simulink model "SiMoDronesMK"  (R2022a)
settings: Solver=FixedStepAuto  StartTime=0.0  StopTime=60  FixedStep=0.005  MaxStep=1e-3  MinStep=5e-5  RelTol=1e-5  AbsTol=1e-5  EnableMultiTasking=on
StopFcn:
  | save log.mat
  | [px4,optitrack,control,simulink]=traite_data_full('log.mat');
  | plot_data;
values from neighbouring files (symbols this model uses):
  aero =     [log.mat]
  drone =     [log.mat]
  dT_px4_udp = 0.02    [SimulationStartupScript.m]    (also in log.mat)
  dT_udp = 0.02    [SimulationStartupScript.m]    (also in log.mat)
  dT_udp_px4 = 0.02    [SimulationStartupScript.m]    (also in log.mat)
  Iload_UAVaxis = [0.00408625  0  0; 0  0.00408625  0; 0  0  8.625e-05]    [log.mat]
  init_state =     [log.mat]
  kpx = 1    [log.mat]
  kvx = 0.35    [log.mat]
  mass = 0.207    [log.mat]
  measure =     [log.mat]
  motor =     [log.mat]
  noisetrigger = 0    [log.mat]
  regul =     [log.mat]
  tdrop = 30    [SimulationStartupScript.m]    (also in log.mat)
  Te = 2e-2    (= 0.02)    [SimulationStartupScript.m]    (also in log.mat)
  th0 = 0.45    [log.mat]
  Ts_px4 = 5e-3    (= 0.005)    [SimulationStartupScript.m]    (also in log.mat)
undefined symbols (not defined in the file or in its folder): DiscIntNeverNeededParam, frame_t, gcbh, sigbuilder_block, sldrt_modeswitch, Standard_Devices, UDP_Protocol
libraries: simulink x11, orocomplib x9, vrlib x5, sldrtlib x4, sharedtransform x3, shared6dofsys x2, sharedutil x1, shared6dof x1, lib_isae_drones x1, simulink_need_slupdate x1, aerolibanimutils x1
(part 1 of 3)
Description:
  | SiMoDronesBE is an simulation environnement for ISAE drones dedicaded at the parrot + px4 bord drone.
settings Model: xpc_rtwmakecfg_data=_xpcnblib__xpcetherlib__xpcether8255xlib__xpcetherGbElib__xpciplib_  ExtModeTrigDuration=300000  Creator=Francois Defay  LastModifiedBy=fades
settings Model: ModifiedHistory=|
  | - Modification of measurement block and visualisation
  | - Some limitations of PWM have been added on the motor
settings SolverCC: AutoScaleAbsTol=off  ZeroCrossAlgorithm=Adaptive  AlgebraicLoopSolver=TrustRegion  AutoInsertRateTranBlk=on  InsertRTBMode=Always
settings DataIOCC: SaveFormat=Array  SaveOutput=off  SignalLogging=off  DSMLogging=off  SaveTime=off  ReturnWorkspaceOutputs=off
settings OptimizationCC: ExpressionDepthLimit=2147483647  LifeSpan=inf
settings DebuggingCC: UnderspecifiedInitializationDetection=Classic  MergeDetectMultiDrivingBlocksExec=none  IgnoredZcDiagnostic=none  SolverPrmCheckMsg=warning  MultiTaskDSMMsg=warning  UnconnectedInputMsg=warning  UnconnectedOutputMsg=warning  UnconnectedLineMsg=warning  AllowSymbolicDim=off  StateNameClashWarn=warning  SFUnexpectedBacktrackingDiag=warning  SFNoUnconditionalDefaultTransitionDiag=warning  SFExecutionAtInitializationDiag=none  SFMachineParentedDataDiag=warning  ArithmeticOperatorsInVariantConditions=warning
settings HardwareCC: ProdBitPerLong=64  ProdHWDeviceType=Intel->x86-64 (Linux 64)  TargetBitPerLong=64  TargetBitPerPointer=64  TargetIntDivRoundTo=Zero  TargetEndianess=LittleEndian  TargetWordSize=64  TargetHWDeviceType=Intel->x86-64
settings ModelReferenceCC: PropagateSignalLabelsOutOfModel=off
settings SFSimCC: SimUseLocalCustomCode=off  CustomCodeUndefinedFunction=UseInterfaceOnly
settings RTWCC: Description=Simulink Desktop Real-Time  SystemTargetFile=sldrt.tlc  TemplateMakefile=sldrt.tmf  RTWUseLocalCustomCode=off  RTWCompilerOptimization=on  DLArmComputeVersion=19.05
settings CodeAppCC: MaxIdLength=95  StateflowObjectComments=on
settings SimulinkDesktopRealTimeCC: TargetLibSuffix=_sldrt.a  TargetPreCompLibLocation=D:\toolbox\sldrt\lib\win64  TargetLangStandard=C89/C90 (ANSI)  SupportVariableSizeSignals=off
settings ConfigComp: CovMetricSettings=dw  CovSaveCumulativeToWorkspaceVar=on  CovSaveSingleToWorkspaceVar=on  CovExternalEMLEnable=off
settings SimscapeCC: SimscapeNormalizeSystem=off
settings ConfigurationSet: Description=SimMechanics 2G

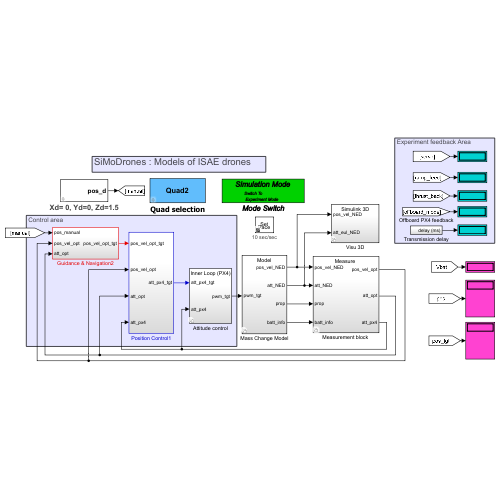
[thumbnail: Simulink's stored preview of the top-level diagram]
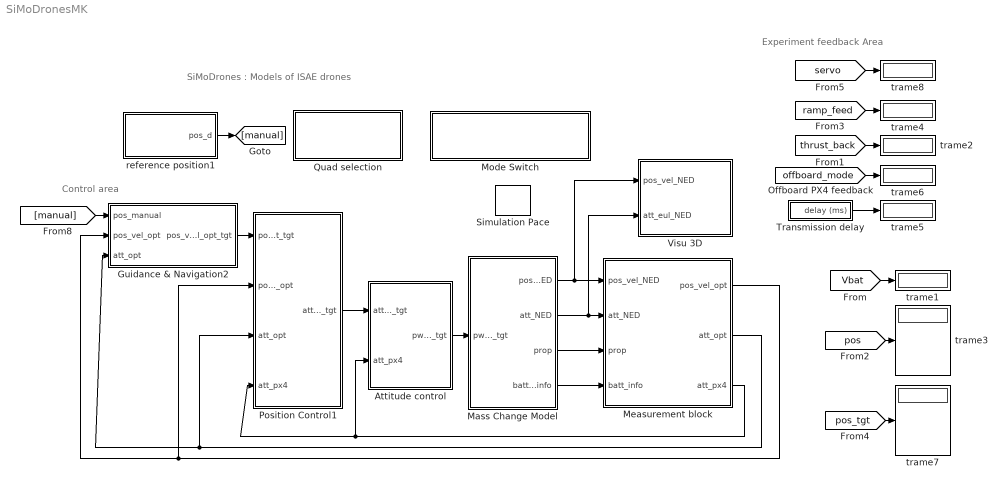
== system SiMoDronesMK ==
  note: Control area
  note: SiMoDrones : Models of ISAE drones
  note: Experiment feedback Area
   trame{1..8} (8 alike) : Display
  Attitude control : Subsystem  Variant=on
  Guidance & Navigation2 : Subsystem
  Mass Change Model : Subsystem  Variant=on
  "Measurement block " : Subsystem  Variant=on
  Mode Switch : Subsystem  LoadFcn=sldrt_modeswitch(gcbh, false)  mask(Mode Switch){}
      settings: OpenFcn=sldrt_modeswitch(gcbh, true)
      mask Display: text(0.5,0.8,'Simulation Mode', 'horizontalAlignment','center');text(0.5,0.5,'_{_{Switch To\newline Experiment Mode}}', 'horizontalAlignment','center','texmode','on');
  Position Control1 : Subsystem
  Quad selection : Subsystem  VariantControl=EXPERIMENT_MODE  mask{quadri_selected=QuadEdu_3}
      mask prompts: quadri_selected "Quadri"
      mask init:
      | assignin('base','quadri_selected', quadri_selected);
      | assignin('base','Quad1', Simulink.Variant('quadri_selected==1'));
      | assignin('base','Quad2', Simulink.Variant('quadri_selected==2'));
      | assignin('base','Quad3', Simulink.Variant('quadri_selected==3'));
      | 
      | if (quadri_selected == 1)
      |     set_param(gcbh, 'MaskDisplay', ...       'text(0.5,0.5,''Quad1'', ''horizontalAlignment'',''center'',''texmode'',''on'')');
      |        'disp(''Quad1'')');
      | elseif (quadri_selected == 2)
      |     set_param(gcbh, 'MaskDisplay', ...
      |        'disp(''MK6'')');
      | elseif (quadri_selected == 3)
      |     set_param(gcbh, 'MaskDisplay', ...
      |        'disp(''Quad2'')');
      | else
      |     set_param(gcbh, 'MaskDisplay', ...
      |        'disp(''No quad'')');
      | end
      mask TypeOptions quadri_selected: QuadEdu_1 | QuadEdu_2 | QuadEdu_3
      mask Display: disp('Quad2')
  Simulation Pace : aerolibanimutils/Simulation Pace  SimulationPace=10  SleepMode=MATLAB Thread  OutputPaceError=off  SampleTime=Te
      settings: AttributesFormatString=%<SimulationPace> sec/sec
  Transmission delay : Subsystem
  Visu 3D : Subsystem  Variant=on
  reference position1 : Subsystem  mask{xd=0, yd=0, zd=1.5}
      mask prompts: xd "X"; yd "Y"; zd "(-Z) Altitude"
      settings: AttributesFormatString=Xd= %<xd>, Yd=%<yd>, Zd=%<zd>
  wires:
  "Measurement block "/2(att_opt) -> Guidance & Navigation2/3(att_opt), Position Control1/3(att_opt)
  Mass Change Model/1(pos_vel_NED) -> "Measurement block "/1(pos_vel_NED), Visu 3D/1(pos_vel_NED)
  Mass Change Model/2(att_NED) -> "Measurement block "/2(att_NED), Visu 3D/2(att_eul_NED)
  Mass Change Model/3(prop) -> "Measurement block "/3(prop)
  Mass Change Model/4(batt_info) -> "Measurement block "/4(batt_info)
  "Measurement block "/1(pos_vel_opt) -> Guidance & Navigation2/2(pos_vel_opt), Position Control1/2(pos_vel_opt)
  Guidance & Navigation2/1(pos_vel_opt_tgt) -> Position Control1/1(pos_vel_opt_tgt)
  Position Control1/1(att_px4_tgt) -> Attitude control/1(att_px4_tgt)
  "Measurement block "/3(att_px4) -> Position Control1/4(att_px4), Attitude control/2(att_px4)
  Attitude control/1(pwm_tgt) -> Mass Change Model/1(pwm_tgt)
  [Vbat] -> " trame1"/1
  [thrust_back] -> " trame2"/1
  [pos] -> " trame3"/1
  [ramp_feed] -> " trame4"/1
  Transmission delay/1(delay (ms)) -> " trame5"/1
  [offboard_mode] -> " trame6"/1
  [pos_tgt] -> " trame7"/1
  [manual] -> Guidance & Navigation2/1(pos_manual)
  [servo] -> " trame8"/1
  reference position1/1(pos_d) -> [manual]

== system SiMoDronesMK/Attitude control ==
  att_px4_tgt : Inport
  att_px4 : Inport  Port=2
  Inner Loop (PX4) : Subsystem  VariantControl=SIMULATION_MODE
  Udp send : Subsystem  VariantControl=EXPERIMENT_MODE
  pwm_tgt : Outport

== system SiMoDronesMK/Guidance & Navigation2 ==
  pos_manual : Inport
  pos_vel_opt : Inport  Port=2
  att_opt : Inport  Port=3
  Bus Selector1 : BusSelector  OutputSignals=x,y,z
  Bus Selector2 : BusSelector  OutputSignals=vx,vy,vz
  Constant : Constant  Value=0
  Demux : Demux  Outputs=3
  Manual Switch3 : ManualSwitch  CurrentSetting=0
  Mux : Mux  Inputs=3
  Mux1 : Mux  Inputs=3
  Mux2 : Mux  Inputs=3
  Signal Builder : Subsystem  Tag=STV Subsys  LoadFcn=sigbuilder_block('load');  StartFcn=sigbuilder_block('start');  StopFcn=sigbuilder_block('stop');  ClipboardFcn=sigbuilder_block('clipboard');  mask(Sigbuilder block){tuvar=[0:10]}
      mask help: Simulink:masks:SigbuilderBlock_MD
      mask init:
      | if ~strcmp(get_param(bdroot(gcbh),'SimulationStatus'),'stopped') tuvar = sigbuilder_block('maskInit'); end
      settings: CopyFcn=sigbuilder_block('copy');  DeleteFcn=sigbuilder_block('delete');  ModelCloseFcn=sigbuilder_block('modelClose');  PreSaveFcn=sigbuilder_block('preSave');  PauseFcn=sigbuilder_block('pause');  ContinueFcn=sigbuilder_block('continue');  NameChangeFcn=sigbuilder_block('namechange');  OpenFcn=sigbuilder_block('open',[285 94 1149 508.25 ]);  CloseFcn=sigbuilder_block('close');
      mask Display: plot(0, 0, 100, 100,[2, 2, 32, 32, 2], [68, 8, 8, 68, 68],[32, 2], [38, 38], [32, 19, 2],[53, 60, 44], [32, 17, 17, 2],[16, 16, 31, 31]);txt = getActiveGroup(gcbh);text(2, 100, txt,'verticalAlignment', 'top');
  Subsystem : Subsystem
  Terminator : Terminator
  Terminator1 : Terminator
  To Workspace1 : ToWorkspace  VariableName=pos_tgt  SampleTime=Te
  To Workspace2 : ToWorkspace  VariableName=vit_tgt  SampleTime=Te
  pos_vel_opt_tgt : Outport  SampleTime=Te
  tag scope: pos_tgt=global
  wires:
  att_opt/1 -> Terminator/1
  Demux/3 -> Subsystem/3(Z_tgt)
  Demux/2 -> Subsystem/2(Y_tgt)
  Demux/1 -> Subsystem/1(X_tgt)
  Constant/1 -> Subsystem/4(Vx_tgt), Subsystem/6(Vz_tgt), Subsystem/5(Vy_tgt)
  Subsystem/1(pos_vel_opt_tgt) -> pos_vel_opt_tgt/1, Bus Selector2/1, Bus Selector1/1
  Mux1/1 -> To Workspace2/1
  Bus Selector2/3 -> Mux1/3  "<vz>"
  Bus Selector2/1 -> Mux1/1  "<vx>"
  Bus Selector2/2 -> Mux1/2  "<vy>"
  Mux/1 -> To Workspace1/1, [pos_tgt]
  Bus Selector1/3 -> Mux/3  "<z>"
  Bus Selector1/1 -> Mux/1  "<x>"
  Bus Selector1/2 -> Mux/2  "<y>"
  pos_manual/1 -> Manual Switch3/1
  Manual Switch3/1 -> Demux/1
  Mux2/1 -> Manual Switch3/2
  Signal Builder/2(Signal 2) -> Mux2/2
  Signal Builder/3(Signal 3) -> Mux2/3
  Signal Builder/1(Signal 1) -> Mux2/1
  pos_vel_opt/1 -> Terminator1/1

== system SiMoDronesMK/Mass Change Model ==
  pwm_tgt : Inport
  Model : Subsystem  VariantControl=SIMULATION_MODE
  Model disabled : Subsystem  VariantControl=EXPERIMENT_MODE
  pos_vel_NED : Outport
  att_NED : Outport  Port=2
  prop : Outport  Port=3
  batt_info : Outport  Port=4

== system SiMoDronesMK/Measurement block  ==
  pos_vel_NED : Inport
  att_NED : Inport  Port=2
  prop : Inport  Port=3
  batt_info : Inport  Port=4
  "Measure " : Subsystem  VariantControl=SIMULATION_MODE
  UDP link + Measure : Subsystem  VariantControl=EXPERIMENT_MODE
  pos_vel_opt : Outport
  att_opt : Outport  Port=2
  att_px4 : Outport  Port=3

== system SiMoDronesMK/Mode Switch ==
  mode : Constant  Value=0

== system SiMoDronesMK/Position Control1 ==
  pos_vel_opt_tgt : Inport
  pos_vel_opt : Inport  Port=2
  att_opt : Inport  Port=3
  att_px4 : Inport  Port=4  SampleTime=Te
  Bus Selector1 : BusSelector  OutputSignals=yaw
  Bus Selector3 : BusSelector  OutputSignals=yaw
  Delay6 : Delay  Commented=through  DelayLength=floor(dT_px4_udp/Te)  InitialCondition=0  SampleTime=Te
  Frame change : Subsystem
  Orocos Mapping : Subsystem
  X control : Subsystem
  Y  control : Subsystem
  Z  control : Subsystem
  psi_opt_tgt : Constant  Value=0
  px4 yaw compensation : Subsystem
  att_px4_tgt : Outport
  wires:
  Orocos Mapping/1(att_px4_tgt) -> att_px4_tgt/1
  px4 yaw compensation/1(yaw_tgt_px4) -> Orocos Mapping/3(yaw)
  pos_vel_opt_tgt/1 -> Y  control/1(pos_vel_opt_tgt), X control/1(pos_vel_opt_tgt), Z  control/1(pos_vel_opt_tgt)
  att_opt/1 -> Bus Selector3/1
  att_px4/1 -> Delay6/1
  Bus Selector3/1 -> px4 yaw compensation/1(psi_opt), Frame change/3(psi)  "<yaw>"
  psi_opt_tgt/1 -> px4 yaw compensation/2(psi_opt_tgt)
  Bus Selector1/1 -> px4 yaw compensation/3(psi_px4)  "<yaw>"
  Delay6/1 -> Bus Selector1/1
  pos_vel_opt/1 -> Y  control/2(pos_vel_opt), X control/2(pos_vel_opt), Z  control/2(pos_vel_opt)
  X control/1(Pitch_tgt) -> Frame change/2(pitch_tgt)
  Y  control/1(Roll_tgt) -> Frame change/1(roll_tgt)
  Z  control/1(Thrust[0..1]) -> Orocos Mapping/4(thrust [0..1])
  Frame change/2(pitch_command) -> Orocos Mapping/2(pitch)
  Frame change/1(roll_command) -> Orocos Mapping/1(roll)

== system SiMoDronesMK/Quad selection ==

== system SiMoDronesMK/Transmission delay ==
  Add : Sum  Inputs=+-
  Data Type Conversion1 : DataTypeConversion  OutDataTypeStr=double  SaturateOnIntegerOverflow=off  LockScale=on
  Gain1 : Gain  Gain=10
  delay (ms) : Outport
  wires:
  [ramp_feed] -> Add/2
  [ramp_out] -> Add/1
  Gain1/1 -> delay (ms)/1
  Add/1 -> Data Type Conversion1/1
  Data Type Conversion1/1 -> Gain1/1

== system SiMoDronesMK/Visu 3D ==
  pos_vel_NED : Inport
  att_eul_NED : Inport  Port=2
  3D disabled : Subsystem  VariantControl=EXPERIMENT_MODE
  Simulink 3D : Subsystem  VariantControl=SIMULATION_MODE

== system SiMoDronesMK/reference position1 ==
  Constant1 : Constant  Value=xd  SampleTime=Te
  Constant2 : Constant  Value=yd  SampleTime=Te
  Constant4 : Constant  Value=zd  SampleTime=Te
  Gain : Gain  Gain=-1
  Mux : Mux  Inputs=3
  pos_d : Outport
  wires:
  Constant1/1 -> Mux/1
  Constant2/1 -> Mux/2
  Constant4/1 -> Gain/1
  Mux/1 -> pos_d/1
  Gain/1 -> Mux/3

== system SiMoDronesMK/Attitude control/Inner Loop (PX4) ==
  att_px4_tgt : Inport
  att_px4 : Inport  Port=2
  Attitude Control Actuators (PID-PX4) : Subsystem  VariantControl=SIMULATION_SIMULINK  mask(PX4 attitude controller){Kp_att=regul.px4.Kp_att, yaw_ff=regul.px4.Yaw_ff, yaw_sp_move_rate=regul.px4.Yaw_move_rate, mc_rate_max=regul.px4.max_rate, Kp_rate=regul.px4.Kp_rate, Ki_rate=regul.px4.Ki_rate, Kd_rate=regul.px4.Kd_rate, ff_rate=regul.px4.ff_rate}
      mask prompts: Kp_att "Proportional gains"; yaw_ff "Yaw feedforward gain"; yaw_sp_move_rate "Yaw move rate"; mc_rate_max "Max rate output (deg/s)"; Kp_rate "Proportional gains"; Ki_rate "Integral gains"; Kd_rate "Derivative gains"; ff_rate "Feedforward gains"
      mask DialogControl Container4 Prompt: MC Attitude control
      mask DialogControl Container12 Prompt: MC Attitude rate control
  Mixer_Quad_X : Subsystem  mask(Mixer Quad X){}
      mask help:
      | Mixer used by a PX4 configured with a Quad X airframe.
      |
      | It takes in the the actuators target (normalized roll, pitch, yaw [-1..1], thrust [0..1]) and mixes them with the Quad X mixer matrix into 4 motors PWM ([0..1]).
      mask DialogControl Container2 Prompt: Parameters
  To Workspace3 : ToWorkspace  Commented=on  VariableName=pwm_target  SampleTime=Te
  pwm_tgt : Outport
  wires:
  att_px4/1 -> Attitude Control Actuators (PID-PX4)/2(att_eul_PX4)
  Attitude Control Actuators (PID-PX4)/1(actuator_target) -> Mixer_Quad_X/1(actuators_tgt)
  Mixer_Quad_X/1(pwm_out) -> pwm_tgt/1, To Workspace3/1
  att_px4_tgt/1 -> Attitude Control Actuators (PID-PX4)/1(att_eul_tgt)

== system SiMoDronesMK/Attitude control/Udp send ==
  att_px4_tgt : Inport
  Bus Selector : BusSelector  OutputSignals=roll,pitch,yaw,thrust
  Constant : Constant  OutDataTypeStr=int16  SampleTime=Te
  Counter Free-Running : simulink/Sources/Counter Free-Running  NumBits=16  tsamp=Te
  Mux : Mux
  To Workspace1 : ToWorkspace  VariableName=att_tgt_px4  SampleTime=Te
  To Workspace3 : ToWorkspace  VariableName=ramp1  SampleTime=Te
  send_udp : Subsystem  Variant=on
  udpSend : MATLAB Function  TreatAsAtomicUnit=on
  tag scope: ramp_out=global
  wires:
  att_px4_tgt/1 -> Bus Selector/1, udpSend/1(att_eul_tgt)
  Constant/1 -> udpSend/2(simulink_out_mode)
  Counter Free-Running/1 -> [ramp_out], To Workspace3/1, udpSend/3(ramp)
  [offboard_mode] -> udpSend/4(simulink_activated)
  udpSend/1(floats) -> send_udp/1(float)
  udpSend/2(integers) -> send_udp/2(Int)
  Mux/1 -> To Workspace1/1
  Bus Selector/4 -> Mux/4  "<thrust>"
  Bus Selector/3 -> Mux/3  "<yaw>"
  Bus Selector/2 -> Mux/2  "<pitch>"
  Bus Selector/1 -> Mux/1  "<roll>"

== system SiMoDronesMK/Guidance & Navigation2/Signal Builder ==
  Demux : Demux  Tag=STV Demux  Outputs=3
      settings: DisplayOption=none
  FromWs : FromWorkspace  Tag=STV FromWs  VariableName=tuvar
      SigBuilderData=|
      | common.afterFinalStr = 'Extrapolate'
      | common.sampleTime = 0
      | dataSet.timeRange = [0 60]
      | dataSet.name = 'Group 1'
      | sbobj.Groups.Name = 'Group 1'
      | sbobj.Groups.Signals(1).Name = 'Signal 1'
      | sbobj.Groups.Signals(1).XData = [0 25 60]
      | sbobj.Groups.Signals(1).YData = [0 0 0]
      | sbobj.Groups.Signals(2).Name = 'Signal 2'
      | sbobj.Groups.Signals(2).XData = [0 5 60]
      | sbobj.Groups.Signals(2).YData = [0 0 0]
      | sbobj.Groups.Signals(3).Name = 'Signal 3'
      | sbobj.Groups.Signals(3).XData = [0 3.45 5 5 15 15 22 22 38 38 45 45 52 55 60]
      | sbobj.Groups.Signals(3).YData = [0 0 -0.75 -0.7 -0.7 -2.15 -2.15 -1.5 -1.5 -2 -2 -1.5 -1.5 0 0]
      | sbobj.Groups.TimeRange = [0 60]
  Signal 1 : Outport  Tag=STV Outport
  Signal 2 : Outport  Tag=STV Outport  Port=2
  Signal 3 : Outport  Tag=STV Outport  Port=3
  wires:
  FromWs/1 -> Demux/1
  Demux/1 -> Signal 1/1
  Demux/2 -> Signal 2/1
  Demux/3 -> Signal 3/1

== system SiMoDronesMK/Guidance & Navigation2/Subsystem ==
  X_tgt : Inport
  Y_tgt : Inport  Port=2
  Z_tgt : Inport  Port=3
  Vx_tgt : Inport  Port=4
  Vy_tgt : Inport  Port=5
  Vz_tgt : Inport  Port=6
  Constant1 : Constant  Value=frame_t.LOCAL_NED
  OROCOS TYPE pos_vel : orocomplib/OROCOS TYPE pos_vel
      settings: SourceProductName=Orocos Component Target
  pos_vel_opt_tgt : Outport
  wires:
  Vx_tgt/1 -> OROCOS TYPE pos_vel/6
  Vz_tgt/1 -> OROCOS TYPE pos_vel/8
  ? -> OROCOS TYPE pos_vel/1
  Vy_tgt/1 -> OROCOS TYPE pos_vel/7
  Z_tgt/1 -> OROCOS TYPE pos_vel/5
  Y_tgt/1 -> OROCOS TYPE pos_vel/4
  X_tgt/1 -> OROCOS TYPE pos_vel/3
  Constant1/1 -> OROCOS TYPE pos_vel/2
  OROCOS TYPE pos_vel/1 -> pos_vel_opt_tgt/1

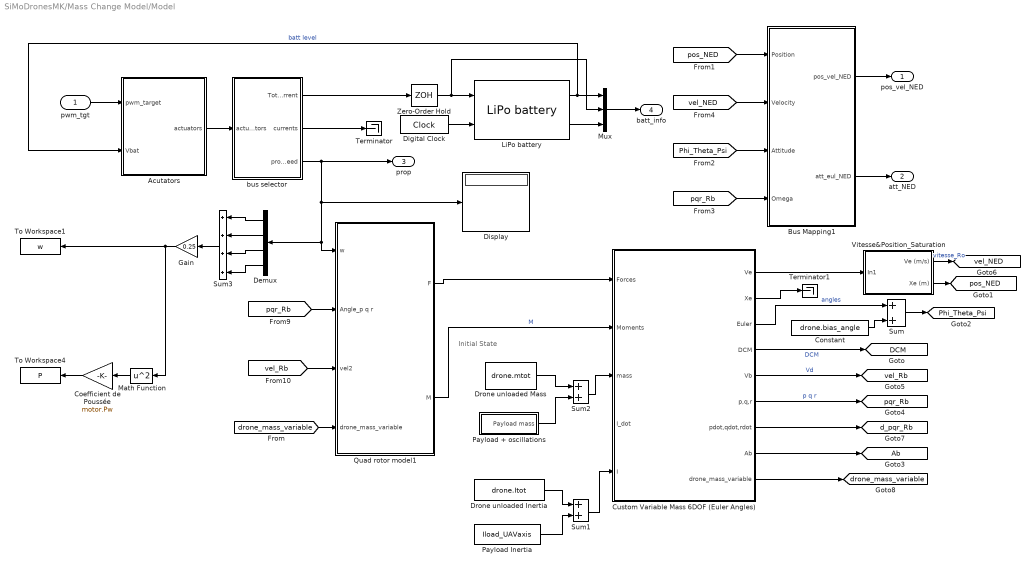
== system SiMoDronesMK/Mass Change Model/Model ==
  note: Initial State
  pwm_tgt : Inport
  Acutators : Subsystem
  Bus Mapping1 : Subsystem
  Coefficient de Poussée : Gain  Gain=motor.Pw
  Constant : Constant  Value=drone.bias_angle
  Custom Variable Mass 6DOF (Euler Angles) : Subsystem  AncestorBlock=shared6dof/6DOF (Euler Angles)  mask(6DOF EoM (Body Axis)){units=Metric (MKS), mtype=Custom Variable, rep=Euler Angles, xme_0=init_state.Pterre0, Vm_0=init_state.Vuvw0, eul_0=init_state.Angles0, pm_0=init_state.pqr0, mass_0=1.0, mass_e=0.5, mass_f=2.0, inertia=eye(3), inertia_e=eye(3), inertia_f=2*eye(3), k_quat=1.0, vre_flag=off, abi_flag=off, aMode=0, xme_statename='', Vm_statename='', eul_statename='', quat_statename='', pm_statename='', mass_statename=''}
      mask prompts: units "shared_aeroblks:sharedaeroblk6dofbody:block6DOFEoMBodyAxisParamUnits"; mtype "shared_aeroblks:sharedaeroblk6dofbody:block6DOFEoMBodyAxisParamMasstype"; rep "shared_aeroblks:sharedaeroblk6dofbody:block6DOFEoMBodyAxisParamRepresentation"; xme_0 "shared_aeroblks:sharedaeroblk6dofbody:block6DOFEoMBodyAxisParamInitialpositionininertialaxesXeYeZe"; Vm_0 "shared_aeroblks:sharedaeroblk6dofbody:block6DOFEoMBodyAxisParamInitialvelocityinbodyaxesUvw"; eul_0 "shared_aeroblks:sharedaeroblk6dofbody:block6DOFEoMBodyAxisParamInitialEulerorientationrollpitchyaw"; pm_0 "shared_aeroblks:sharedaeroblk6dofbody:block6DOFEoMBodyAxisParamInitialbodyrotationratespqr"; mass_0 "shared_aeroblks:sharedaeroblk6dofbody:block6DOFEoMBodyAxisParamInitialmass"; mass_e "shared_aeroblks:sharedaeroblk6dofbody:block6DOFEoMBodyAxisParamEmptymass"; mass_f "shared_aeroblks:sharedaeroblk6dofbody:block6DOFEoMBodyAxisParamFullmass"; inertia "shared_aeroblks:sharedaeroblk6dofbody:block6DOFEoMBodyAxisParamInertia"; inertia_e "shared_aeroblks:sharedaeroblk6dofbody:block6DOFEoMBodyAxisParamEmptyinertiamatrix"; inertia_f "shared_aeroblks:sharedaeroblk6dofbody:block6DOFEoMBodyAxisParamFullinertiamatrix"; k_quat "shared_aeroblks:sharedaeroblk6dofbody:block6DOFEoMBodyAxisParamGainforquaternionnormalization"; vre_flag "shared_aeroblks:sharedaeroblk6dofbody:block6DOFEoMBodyAxisParamIncludemassflowrelativevelocity"; abi_flag "shared_aeroblks:sharedaeroblk6dofbody:inertialAccelFlag"; xme_statename "shared_aeroblks:sharedaeroblk6dofbody:block6DOFEoMStateNamePosition"; Vm_statename "shared_aeroblks:sharedaeroblk6dofbody:block6DOFEoMStateNameVelocity"; eul_statename "shared_aeroblks:sharedaeroblk6dofbody:block6DOFEoMStateNameEulerAngles"; quat_statename "shared_aeroblks:sharedaeroblk6dofbody:block6DOFEoMStateNameQuaternions"; pm_statename "shared_aeroblks:sharedaeroblk6dofbody:block6DOFEoMStateNameRotationRates"; mass_statename "shared_aeroblks:sharedaeroblk6dofbody:block6DOFEoMStateNameMass"
      mask help: shared_aeroblks:sharedaeroblk6dofbody:block6DOFEoMBodyAxisDesc
      mask init:
      | if aerosharedtest(gcb)
      |     ports=aerosharedicon('shared6dofbody','icon');
      | else
      |     ports=sharedautoicon('shared6dofbody','icon');
      | end
      mask Help: eval('aerosharedhelp(''custom_variable_mass_sixdof_euler_angles'')');
      mask TypeOptions units: shared_aeroblks:sharedaeroblk6dofbody:block6DOFEoMBodyAxisParamComboMetricMKS | shared_aeroblks:sharedaeroblk6dofbody:block6DOFEoMBodyAxisParamComboEnglishVelocityinfts | shared_aeroblks:sharedaeroblk6dofbody:block6DOFEoMBodyAxisParamComboEnglishVelocityinkts
      mask TypeOptions mtype: shared_aeroblks:sharedaeroblk6dofbody:block6DOFEoMBodyAxisParamComboFixed | shared_aeroblks:sharedaeroblk6dofbody:block6DOFEoMBodyAxisParamComboSimpleVariable | shared_aeroblks:sharedaeroblk6dofbody:block6DOFEoMBodyAxisParamComboCustomVariable
      mask Callback mtype:
      | if aerosharedtest(gcb) && builtin('license','test','aerospace_blockset')
      |     aerosharedicon('shared6dofbody');
      | else
      |     sharedautoicon('shared6dofbody');
      | end
      mask TypeOptions rep: shared_aeroblks:sharedaeroblk6dofbody:block6DOFEoMBodyAxisParamComboEulerAngles | shared_aeroblks:sharedaeroblk6dofbody:block6DOFEoMBodyAxisParamComboQuaternion
      mask Callback rep:
      | if aerosharedtest(gcb) && builtin('license','test','aerospace_blockset')
      |     aerosharedicon('shared6dofbody');
      | else
      |     sharedautoicon('shared6dofbody');
      | end
      mask DialogControl Container4 Prompt: shared_aeroblks:sharedaeroblk6dofbody:block6DOFEoMParamTab
      mask DialogControl units Prompt: Units:
      mask DialogControl mtype Prompt: Mass type:
      mask DialogControl rep Prompt: Representation:
      mask DialogControl xme_0 Prompt: Initial position in inertial axes [Xe,Ye,Ze]:
      mask DialogControl Vm_0 Prompt: Initial velocity in body axes [U,v,w]:
      mask DialogControl eul_0 Prompt: Initial Euler orientation [roll, pitch, yaw]:
      mask DialogControl pm_0 Prompt: Initial body rotation rates [p,q,r]:
      mask DialogControl mass_0 Prompt: Initial mass:
      mask DialogControl mass_e Prompt: Empty mass:
      mask DialogControl mass_f Prompt: Full mass:
      mask DialogControl inertia Prompt: Inertia:
      mask DialogControl inertia_e Prompt: Empty inertia matrix:
      mask DialogControl inertia_f Prompt: Full inertia matrix:
      mask DialogControl k_quat Prompt: Gain for quaternion normalization:
      mask DialogControl vre_flag Prompt: Include mass flow relative velocity
      mask DialogControl abi_flag Prompt: Include inertial acceleration
      mask DialogControl Container6 Prompt: shared_aeroblks:sharedaeroblk6dofbody:block6DOFEoMStateAttributesTab
      mask DialogControl Container7 Prompt: shared_aeroblks:sharedaeroblk6dofbody:block6DOFEoMStateNamesGroup
      mask DialogControl xme_statename Prompt: Position: e.g., {'Xe', 'Ye', 'Ze'}
      mask DialogControl Vm_statename Prompt: Velocity: e.g., {'U', 'v', 'w'}
      mask DialogControl eul_statename Prompt: Euler rotation angles: e.g., {'phi', 'theta', 'psi'}
      mask DialogControl quat_statename Prompt: Quaternion vector: e.g., {'qr', 'qi', 'qj', 'qk'}
      mask DialogControl pm_statename Prompt: Body rotation rates: e.g., {'p', 'q', 'r'}
      mask DialogControl mass_statename Prompt: Mass: e.g., 'mass'
      mask Display:
      | port_label(ports(1).type,ports(1).port,ports(1).txt,'texmode','on');
      | port_label(ports(2).type,ports(2).port,ports(2).txt,'texmode','on');
      | port_label(ports(3).type,ports(3).port,ports(3).txt,'texmode','on');
      | port_label(ports(4).type,ports(4).port,ports(4).txt,'texmode','on');
      | port_label(ports(5).type,ports(5).port,ports(5).txt,'texmode','on');
      | port_label(ports(6).type,ports(6).port,ports(6).txt,'texmode','on');
      | port_label(ports(7).type,ports(7).port,ports(7).txt,'texmode','on');
      | port_label(ports(8).type,ports(8).port,ports(8).txt,'texmode','on');
      | port_label(ports(9).type,ports(9).port,ports(9).txt,'texmode','on');
      | port_label(ports(10).type,ports(10).port,ports(10).txt,'texmode','on');
      | port_label(ports(11).type,ports(11).port,ports(11).txt,'texmode','on');
      | port_label(ports(12).type,ports(12).port,ports(12).txt,'texmode','on');
      | port_label(ports(13).type,ports(13).port,ports(13).txt,'texmode','on');
      | port_label(ports(14).type,ports(14).port,ports(14).txt,'texmode','on');
      | port_label(ports(15).type,ports(15).port,ports(15).txt,'texmode','on');
      | port_label(ports(16).type,ports(16).port,ports(16).txt,'texmode','on');
      | port_label(ports(17).type,ports(17).port,ports(17).txt,'texmode','on');
  Demux : Demux
  Digital Clock : DigitalClock  SampleTime=Te
  Display : Display
  Drone unloaded Inertia : Constant  Value=drone.Itot
  Drone unloaded Mass : Constant  Value=drone.mtot
  Gain : Gain  Gain=0.25
  LiPo battery : lib_isae_drones/LiPo battery  nb_elements=batt.nb_element  capacity=batt.capacity  initial_voltage=batt.initial_voltage  internal_resistance=batt.internal_resistance
      settings: SourceProductName=ISAE drones
  Math Function : Math  Operator=square  SignedPower=on
  Mux : Mux  Inputs=3
  "Payload + oscillations " : Subsystem
  Payload Inertia : Constant  Value=Iload_UAVaxis
  Quad rotor model1 : Subsystem  mask{Pw=motor.Pw, L=drone.length_arm, Mw=motor.Mw, mtot=drone.mtot, rho=aero.rho, S_drag_uvw=aero.S_trainee_uvw, C_drag=aero.C_trainee, g=aero.g, C_trainee=0, S_trainee_pqr=0}
      mask prompts: Pw "Thrust factor"; L "Length of the arm"; Mw "Torque coefficient"; mtot "Total mass"; rho "Air density"; S_drag_uvw "Drag Surface"; C_drag "Drag coefficient"; g "Gravity constant"; C_trainee "rotationnal drag coef"; S_trainee_pqr "rotationnal drag surface"
  Sum : Sum
  Sum1 : Sum
  Sum2 : Sum
  Sum3 : Sum  Inputs=++++
  Terminator : Terminator
  Terminator1 : Terminator
  To Workspace1 : ToWorkspace  VariableName=w  SampleTime=Te
  To Workspace4 : ToWorkspace  VariableName=P  SampleTime=Te
  Vitesse&Position_Saturation : Subsystem
  Zero-Order Hold : ZeroOrderHold  SampleTime=Te
  bus selector : Subsystem
  pos_vel_NED : Outport
  att_NED : Outport  Port=2
  prop : Outport  Port=3
  batt_info : Outport  Port=4
  tag scope: Ab=global, DCM=global, Phi_Theta_Psi=global, d_pqr_Rb=global, drone_mass_variable=global, pos_NED=global, pqr_Rb=global, vel_NED=global, vel_Rb=global
  wires:
  Vitesse&Position_Saturation/1(Ve (m/s)) -> [vel_NED]  "vitesse_Ro"
  Custom Variable Mass 6DOF (Euler Angles)/8(Ab) -> [Ab]
  Custom Variable Mass 6DOF (Euler Angles)/5(Vb) -> [vel_Rb]  "Vd"
  Custom Variable Mass 6DOF (Euler Angles)/4(DCM) -> [DCM]  "DCM"
  Custom Variable Mass 6DOF (Euler Angles)/3(Euler) -> Sum/1  "angles"
  Custom Variable Mass 6DOF (Euler Angles)/1(Ve) -> Vitesse&Position_Saturation/1(In1)
  Custom Variable Mass 6DOF (Euler Angles)/2(Xe) -> Terminator1/1
  Custom Variable Mass 6DOF (Euler Angles)/6(p,q,r) -> [pqr_Rb]  "p q r"
  Custom Variable Mass 6DOF (Euler Angles)/7(pdot,qdot,rdot) -> [d_pqr_Rb]
  bus selector/3(prop speed) -> prop/1, Demux/1, Quad rotor model1/1(w), Display/1
  [pqr_Rb] -> Quad rotor model1/2(Angle_p q r)
  Mux/1 -> batt_info/1
  bus selector/2(currents) -> Terminator/1
  bus selector/1(Total current) -> Zero-Order Hold/1
  LiPo battery/2 -> Mux/3
  Digital Clock/1 -> LiPo battery/2
  LiPo battery/1 -> Acutators/2(Vbat), Mux/1  "batt level"
  pwm_tgt/1 -> Acutators/1(pwm_target)
  Acutators/1(actuators) -> bus selector/1(actuators)
  [pos_NED] -> Bus Mapping1/1(Position)
  [vel_NED] -> Bus Mapping1/2(Velocity)
  [pqr_Rb] -> Bus Mapping1/4(Omega)
  [Phi_Theta_Psi] -> Bus Mapping1/3(Attitude)
  Bus Mapping1/2(att_eul_NED) -> att_NED/1
  Bus Mapping1/1(pos_vel_NED) -> pos_vel_NED/1
  [vel_Rb] -> Quad rotor model1/3(vel2)
  Sum/1 -> [Phi_Theta_Psi]
  Constant/1 -> Sum/2
  Vitesse&Position_Saturation/2(Xe (m)) -> [pos_NED]
  Quad rotor model1/1(F) -> Custom Variable Mass 6DOF (Euler Angles)/1(Forces)
  Quad rotor model1/2(M) -> Custom Variable Mass 6DOF (Euler Angles)/2(Moments)  "M"
  Drone unloaded Mass/1 -> Sum2/1
  Custom Variable Mass 6DOF (Euler Angles)/9(drone_mass_variable) -> [drone_mass_variable]
  Drone unloaded Inertia/1 -> Sum1/1
  Sum1/1 -> Custom Variable Mass 6DOF (Euler Angles)/5(I)
  Sum2/1 -> Custom Variable Mass 6DOF (Euler Angles)/3(mass)
  "Payload + oscillations "/1(Payload mass) -> Sum2/2
  Payload Inertia/1 -> Sum1/2
  [drone_mass_variable] -> Quad rotor model1/4(drone_mass_variable)
  Demux/1 -> Sum3/1
  Demux/2 -> Sum3/2
  Demux/3 -> Sum3/3
  Demux/4 -> Sum3/4
  Sum3/1 -> Gain/1
  Gain/1 -> To Workspace1/1, Math Function/1
  Math Function/1 -> Coefficient de Poussée/1
  Coefficient de Poussée/1 -> To Workspace4/1
  Zero-Order Hold/1 -> Mux/2, LiPo battery/1

== system SiMoDronesMK/Mass Change Model/Model disabled ==

== system SiMoDronesMK/Measurement block /Measure  ==
  pos_vel_NED : Inport
  att_NED : Inport  Port=2
  prop : Inport  Port=3
  batt_info : Inport  Port=4
  Band-Limited White Noise4 : simulink/Sources/Band-Limited White Noise  Cov=[measure.noise_power_propellers]  Ts=Te  seed=[23341]
  Clock : Clock
  Delay2 : Delay  DelayLength=floor(dT_px4_udp/Te)  InitialCondition=0  SampleTime=Te
  Demux : Demux  Outputs=2
  Sum4 : Sum  Inputs=++|
  Terminator : Terminator
  To Workspace5 : ToWorkspace  VariableName=batt_info  SampleTime=Te
  To Workspace6 : ToWorkspace  Commented=on  VariableName=prop_mes  SampleTime=Te
  To Workspace8 : ToWorkspace  VariableName=time_simu  SampleTime=Te
  Zero-Order Hold8 : ZeroOrderHold  SampleTime=0.5
  optitrack : Subsystem
  px4 : Subsystem
  pos_vel_opt : Outport
  att_opt : Outport  Port=2
  att_px4 : Outport  Port=3
  tag scope: Vbat=global, pos=global
  wires:
  optitrack/2(att_eul_optitrack) -> att_opt/1
  optitrack/1(pos_vel_optitrack) -> pos_vel_opt/1
  pos_vel_NED/1 -> Demux/1, optitrack/1(pos_vel_NED)
  px4/1(att_eul_px4) -> att_px4/1
  Delay2/1 -> Sum4/2
  Zero-Order Hold8/1 -> [Vbat], To Workspace5/1
  Clock/1 -> To Workspace8/1
  batt_info/1 -> Zero-Order Hold8/1
  att_NED/1 -> px4/1(att_eul_NED), optitrack/2(att_eul_NED)
  prop/1 -> Delay2/1
  Band-Limited White Noise4/1 -> Sum4/1
  Sum4/1 -> To Workspace6/1, Terminator/1  "prop_mes"
  Demux/1 -> [pos]

== system SiMoDronesMK/Measurement block /UDP link + Measure ==
  Mesure : Subsystem
  UDP link : Subsystem
  pos_vel_opt : Outport
  att_px4 : Outport  Port=2
  att_opt : Outport  Port=3
  wires:
  Mesure/1(pos_vel_optitrack) -> pos_vel_opt/1
  Mesure/2(att_eul_optitrack) -> att_opt/1
  Mesure/3(att_eul_px4_) -> att_px4/1
  UDP link/2(att_eul_optitrack) -> Mesure/2(att_eul_opti)
  UDP link/1(pos_vel_optitrack) -> Mesure/1(pos_vel_opti)
  UDP link/3(att_eul_px4) -> Mesure/3(att_eul_px4)

== system SiMoDronesMK/Position Control1/Frame change ==
  roll_tgt : Inport
  pitch_tgt : Inport  Port=2
  psi : Inport  Port=3
  Add : Sum
  Add1 : Sum
  Gain1 : Gain  Gain=-1
  Product{,1..3} (4 alike) : Product
  Saturation : Saturate  UpperLimit=0.3  LowerLimit=-0.3
  Saturation1 : Saturate  UpperLimit=0.3  LowerLimit=-0.3
  Trigonometric Function : Trigonometry
  Trigonometric Function1 : Trigonometry  Operator=cos
  Trigonometric Function2 : Trigonometry
  Trigonometric Function3 : Trigonometry  Operator=cos
  roll_command : Outport
  pitch_command : Outport  Port=2
  wires:
  Gain1/1 -> Product/1
  Add1/1 -> Saturation1/1
  Product3/1 -> Add1/2
  Trigonometric Function1/1 -> Product3/1
  Product2/1 -> Add1/1
  Trigonometric Function2/1 -> Product2/1
  psi/1 -> Trigonometric Function/1, Trigonometric Function3/1, Trigonometric Function2/1, Trigonometric Function1/1
  Add/1 -> Saturation/1
  Product1/1 -> Add/2
  pitch_tgt/1 -> Product1/2, Product2/2
  Trigonometric Function3/1 -> Product1/1
  Product/1 -> Add/1
  roll_tgt/1 -> Product/2, Product3/2
  Trigonometric Function/1 -> Gain1/1
  Saturation/1 -> pitch_command/1
  Saturation1/1 -> roll_command/1

== system SiMoDronesMK/Position Control1/Orocos Mapping ==
  roll : Inport
  pitch : Inport  Port=2
  yaw : Inport  Port=3
  thrust [0..1] : Inport  Port=4
  Constant : Constant  Value=0  SampleTime=Te
  Constant1 : Constant  Value=0  SampleTime=Te
  Digital Clock : DigitalClock  SampleTime=Te
  OROCOS TYPE attitude_target : orocomplib/OROCOS TYPE attitude_target
      settings: SourceProductName=Orocos Component Target
  att_px4_tgt : Outport
  wires:
  Digital Clock/1 -> OROCOS TYPE attitude_target/1
  Constant1/1 -> OROCOS TYPE attitude_target/2
  Constant/1 -> OROCOS TYPE attitude_target/7, OROCOS TYPE attitude_target/8, OROCOS TYPE attitude_target/6
  OROCOS TYPE attitude_target/1 -> att_px4_tgt/1
  roll/1 -> OROCOS TYPE attitude_target/3
  pitch/1 -> OROCOS TYPE attitude_target/4
  yaw/1 -> OROCOS TYPE attitude_target/5
  thrust [0..1]/1 -> OROCOS TYPE attitude_target/9

== system SiMoDronesMK/Position Control1/X control ==
  pos_vel_opt_tgt : Inport
  pos_vel_opt : Inport  Port=2
  Bus Selector : BusSelector  OutputSignals=x
  Bus Selector1 : BusSelector  OutputSignals=x,vx
  Controller1 : Subsystem
  Pitch_tgt : Outport
  wires:
  Bus Selector1/1 -> Controller1/2(X)  "<x>"
  Controller1/1(Theta_tgt) -> Pitch_tgt/1
  pos_vel_opt_tgt/1 -> Bus Selector/1
  pos_vel_opt/1 -> Bus Selector1/1
  Bus Selector/1 -> Controller1/1(Xr)  "<x>"
  Bus Selector1/2 -> Controller1/3(Vx)  "<vx>"

== system SiMoDronesMK/Position Control1/Y  control ==
  pos_vel_opt_tgt : Inport
  pos_vel_opt : Inport  Port=2
  Bus Selector : BusSelector  OutputSignals=y
  Bus Selector1 : BusSelector  OutputSignals=y,vy
  Controller : Subsystem
  Roll_tgt : Outport
  tag scope: Y=global
  wires:
  pos_vel_opt/1 -> Bus Selector1/1
  pos_vel_opt_tgt/1 -> Bus Selector/1
  Controller/1(Roll_tgt) -> Roll_tgt/1
  Bus Selector1/1 -> [Y], Controller/2(Y)  "<y>"
  Bus Selector1/2 -> Controller/3(Vy)  "<vy>"
  Bus Selector/1 -> Controller/1(Yr)  "<y>"

== system SiMoDronesMK/Position Control1/Z  control ==
  pos_vel_opt_tgt : Inport
  pos_vel_opt : Inport  Port=2
  Bus Selector : BusSelector  OutputSignals=z
  Bus Selector1 : BusSelector  OutputSignals=z,vz
  Controller : Subsystem
  Thrust[0..1] : Outport
  wires:
  pos_vel_opt/1 -> Bus Selector1/1
  pos_vel_opt_tgt/1 -> Bus Selector/1
  ? -> Thrust[0..1]/1
  Bus Selector1/1 -> ?  "<z>"
  Bus Selector1/2 -> ?  "<vz>"
  Bus Selector/1 -> ?  "<z>"

== system SiMoDronesMK/Position Control1/px4 yaw compensation ==
  psi_opt : Inport
  psi_opt_tgt : Inport  Port=2
  psi_px4 : Inport  Port=3
  Sum : Sum  Inputs=|+-
  Sum1 : Sum  Inputs=++|
  yaw_tgt_px4 : Outport  SampleTime=Te
  wires:
  Sum/1 -> Sum1/1
  psi_opt_tgt/1 -> Sum1/2
  psi_opt/1 -> Sum/2
  psi_px4/1 -> Sum/1
  Sum1/1 -> yaw_tgt_px4/1

== system SiMoDronesMK/Visu 3D/3D disabled ==

== system SiMoDronesMK/Visu 3D/Simulink 3D ==
  pos_vel_NED : Inport
  att_eul_NED : Inport  Port=2
  Coordinate Transformations : Subsystem
  VR Sink : vrlib/VR Sink  InstantiateOnLoad=on  SampleTime=0.1  ViewEnable=on  RemoteChange=off  RemoteView=off  FieldsWritten=Camera_Follow.rotation.4.1.1.double#Camera_Follow.translation.3.1.1.double#Copter.rotation.4.1.1.double#Copter.translation.3.1.1.double  WorldFileName=Visu/ArduCopter.wrl  WorldDescription=VR Arducopter  AutoView=off  VideoDimensions=[]  AllowVariableSize=off
  wires:
  Coordinate Transformations/4(position) -> VR Sink/4
  Coordinate Transformations/3(orientation) -> VR Sink/3
  Coordinate Transformations/2(CameraFollowTranslation) -> VR Sink/2
  Coordinate Transformations/1(CameraFollowRotation) -> VR Sink/1
  att_eul_NED/1 -> Coordinate Transformations/1(att_eul)
  pos_vel_NED/1 -> Coordinate Transformations/2(pos_vel)

== system SiMoDronesMK/Attitude control/Inner Loop (PX4)/Attitude Control Actuators (PID-PX4) ==
  att_eul_tgt : Inport  SampleTime=Ts_px4
  att_eul_PX4 : Inport  Port=2
  Bus Selector4 : BusSelector  OutputSignals=roll,pitch,yaw,thrust
  Constant3 : Constant  Value=0  OutDataTypeStr=Inherit: Inherit via back propagation  SampleTime=-1
  Delay4 : Delay  DelayLength=floor(dT_udp_px4/Te)
  Digital Clock : DigitalClock  SampleTime=-1
  Display : Display
  Mux : Mux  Inputs=8
  Mux1 : Mux
  OROCOS TYPE actuator_control_target : orocomplib/OROCOS TYPE actuator_control_target
      settings: SourceProductName=Orocos Component Target
  Régulations : Subsystem
  Saturation : Saturate  UpperLimit=motor.pwm_max  LowerLimit=motor.pwm_min
  To Workspace1 : ToWorkspace  VariableName=att_tgt_px4  SampleTime=Te
  actuator_target : Outport  SampleTime=Ts_px4
  wires:
  Régulations/2(Out2) -> Mux/2  "control2"
  Régulations/4(thrust) -> Mux/4  "control4"
  att_eul_PX4/1 -> Régulations/5(att_eul)
  Delay4/1 -> To Workspace1/1
  Saturation/1 -> Mux1/4, Régulations/4(thrust_d)
  Mux1/1 -> Display/1, Delay4/1
  att_eul_tgt/1 -> Bus Selector4/1  "att_target_Rb"
  Bus Selector4/4 -> Saturation/1  "<thrust>"
  Bus Selector4/3 -> Mux1/3, Régulations/3(In3)  "<yaw>"
  Bus Selector4/2 -> Mux1/2, Régulations/2(In2)  "<pitch>"
  Bus Selector4/1 -> Mux1/1, Régulations/1(In1)  "<roll>"
  Régulations/1(Out1) -> Mux/1  "control1"
  Régulations/3(Out3) -> Mux/3  "control3"
  Mux/1 -> OROCOS TYPE actuator_control_target/2
  OROCOS TYPE actuator_control_target/1 -> actuator_target/1
  Digital Clock/1 -> OROCOS TYPE actuator_control_target/1
  Constant3/1 -> Mux/5, Mux/6, Mux/7, Mux/8

== system SiMoDronesMK/Attitude control/Inner Loop (PX4)/Mixer_Quad_X ==
  actuators_tgt : Inport  OutDataTypeStr=Bus: actuator_control_target
  Bus Selector : BusSelector  OutputSignals=controls
  Demux : Demux  Outputs=8
  Demux1 : Demux
  Gain : Gain  Gain=[0.707107 0.707107 -1 1;-0.707107 0.707107 1 1; -0.707107 -0.707107 -1 1; 0.707107 -0.707107 1 1]  Multiplication=Matrix(K*u) (u vector)
  Ground : Ground
  Mux : Mux  Inputs=8
  Mux3 : Mux
  Saturation1 : Saturate  UpperLimit=1  LowerLimit=-1
  Saturation2 : Saturate  UpperLimit=1  LowerLimit=-1
  Saturation3 : Saturate  UpperLimit=1  LowerLimit=-1
  Saturation4 : Saturate  UpperLimit=1  LowerLimit=0
  Terminator{,1..3} (4 alike) : Terminator
  pwm_out : Outport  BusOutputAsStruct=on
  wires:
  Mux3/1 -> Gain/1
  Gain/1 -> Demux1/1
  actuators_tgt/1 -> Bus Selector/1
  Bus Selector/1 -> Demux/1  "<controls>"
  Demux/1 -> Saturation3/1
  Demux/4 -> Saturation4/1
  Demux/2 -> Saturation1/1
  Demux/3 -> Saturation2/1
  Demux/5 -> Terminator/1
  Demux/6 -> Terminator1/1
  Demux/7 -> Terminator2/1
  Demux/8 -> Terminator3/1
  Saturation3/1 -> Mux3/1
  Saturation1/1 -> Mux3/2
  Saturation2/1 -> Mux3/3
  Saturation4/1 -> Mux3/4
  Demux1/4 -> Mux/4
  Demux1/2 -> Mux/2
  Demux1/1 -> Mux/1
  Demux1/3 -> Mux/3
  Mux/1 -> pwm_out/1
  Ground/1 -> Mux/8, Mux/5, Mux/6, Mux/7

== system SiMoDronesMK/Attitude control/Udp send/send_udp ==
  note: 1) Add Subsystem or Model blocks as valid variant choices.
      | 2) You cannot connect blocks at this level. At simulation, connectivity is automatically
      | determined, based on the active variant and port name matching.
  float : Inport
  Int : Inport  Port=2
  QUADRI_EDU1 : Subsystem  VariantControl=Quad1
  QUADRI_EDU2 : Subsystem  VariantControl=Quad2
  QUADRI_EDU3 : Subsystem  VariantControl=Quad3

== system SiMoDronesMK/Mass Change Model/Model/Acutators ==
  pwm_target : Inport
  Vbat : Inport  Port=2
  Data Type Conversion{,1..3} (4 alike) : DataTypeConversion  SaturateOnIntegerOverflow=off  RndMeth=Floor
  Demux : Demux  Outputs=8
  Motor1 : Subsystem
  Motor2 : Subsystem
  Motor3 : Subsystem
  Motor4 : Subsystem
  Subsystem : Subsystem
      mask Display: disp('Bus definitaion')
  Terminator{,1..3} (4 alike) : Terminator
  actuators : Outport
  wires:
  pwm_target/1 -> Demux/1
  Motor4/4(current) -> Subsystem/16(In16)
  Motor4/3(Torque) -> Subsystem/15(In15)
  Motor4/2(Thrust) -> Subsystem/14(In14)
  Motor4/1(speed) -> Subsystem/13(In12)
  Motor3/4(current) -> Subsystem/12(In11)
  Motor3/3(Torque) -> Subsystem/11(In10)
  Motor3/2(Thrust) -> Subsystem/10(In9)
  Motor3/1(speed) -> Subsystem/9(In8)
  Motor2/4(current) -> Subsystem/8(In7)
  Motor2/3(Torque) -> Subsystem/7(In6)
  Motor2/2(Thrust) -> Subsystem/6(In5)
  Motor2/1(speed) -> Subsystem/5(In4)
  Motor1/4(current) -> Subsystem/4(In13)
  Motor1/3(Torque) -> Subsystem/3(In3)
  Motor1/2(Thrust) -> Subsystem/2(In2)
  Motor1/1(speed) -> Subsystem/1(In1)
  Subsystem/1(actuators) -> actuators/1
  Data Type Conversion/1 -> Motor1/1(PWM)
  Vbat/1 -> Motor1/2(Vbat), Motor2/2(Vbat), Motor3/2(Vbat), Motor4/2(Vbat)
  Data Type Conversion3/1 -> Motor4/1(PWM)
  Data Type Conversion2/1 -> Motor3/1(PWM)
  Data Type Conversion1/1 -> Motor2/1(PWM)
  Demux/7 -> Terminator2/1
  Demux/6 -> Terminator1/1
  Demux/5 -> Terminator/1
  Demux/8 -> Terminator3/1
  Demux/2 -> Data Type Conversion1/1
  Demux/3 -> Data Type Conversion2/1
  Demux/4 -> Data Type Conversion3/1
  Demux/1 -> Data Type Conversion/1

== system SiMoDronesMK/Mass Change Model/Model/Bus Mapping1 ==
  Position : Inport
  Velocity : Inport  Port=2
  Attitude : Inport  Port=3
  Omega : Inport  Port=4
  Mux : Mux  Inputs=2
  Mux1 : Mux  Inputs=2
  pos_vel_NED : Outport
  att_eul_NED : Outport  Port=2
  wires:
  Mux1/1 -> att_eul_NED/1
  Mux/1 -> pos_vel_NED/1
  Velocity/1 -> Mux/2
  Position/1 -> Mux/1
  Omega/1 -> Mux1/2
  Attitude/1 -> Mux1/1

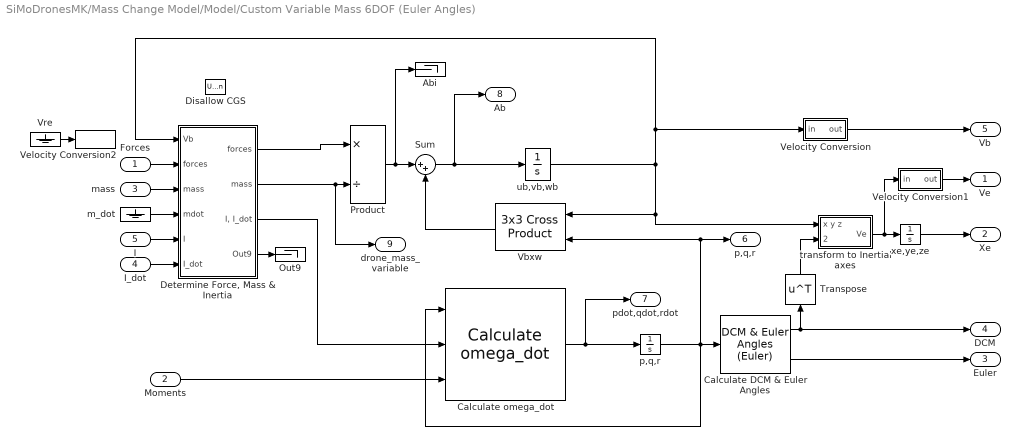
== system SiMoDronesMK/Mass Change Model/Model/Custom Variable Mass 6DOF (Euler Angles) ==
  Forces : Inport  Unit=N  PortDimensions=3
  Moments : Inport  Port=2  Unit=N*m  PortDimensions=3
  mass : Inport  Port=3  Unit=kg
  I_dot : Inport  Port=4  Unit=kg*m^2/s  PortDimensions=[3 3]
  I : Inport  Port=5  Unit=kg*m^2  PortDimensions=[3 3]
  Abi : Terminator
  Calculate DCM & Euler Angles : shared6dofsys/DCM & Euler Angles (Euler)  aMode=aMode
      settings: SourceProductBaseCode=AE,PW,DR,MT,VE
  Calculate omega_dot : shared6dofsys/Calculate omega_dot  aMode=aMode
      settings: SourceProductBaseCode=AE,PW,DR,MT,VE
  "Determine Force, Mass & Inertia" : Subsystem  AncestorBlock=aerolibobsolete/Mass & Inertia (custom)  mask(Mass & Inertia (custom)){}
      mask init:
      | aeroicon('aeroblk');
  Disallow CGS : UnitConfiguration  UnitSystemsStr=English,SI,SI (extended)  AllowAllUnitSystems=off
  Out9 : Terminator
  Product : Product  Inputs=*/  SaturateOnIntegerOverflow=on  OutDataTypeStr=Inherit: Same as first input
  Sum : Sum  Inputs=|++  SaturateOnIntegerOverflow=on
  Transpose : Math  Operator=transpose  SignedPower=on
  Vbxw : sharedutil/3x3 Cross Product  aMode=aMode
      settings: SourceProductBaseCode=AE,PW,DR,MT,VE
  Velocity Conversion : Subsystem
  Velocity Conversion1 : Subsystem
  Velocity Conversion2 : shared6dof/6DOF (Euler Angles)/Velocity Conversion2  SystemSampleTime=-1  VariantActivationTime=update diagram  Latency=0  AutoFrameSizeCalculation=off
      settings: SourceProductBaseCode=AE,PW,DR,MT,VE
  Vre : Ground
  m_dot : Ground
  "p,q,r " : Integrator  InitialCondition=pm_0  ContinuousStateAttributes=pm_statename
  "transform to Inertial axes " : Subsystem  mask(Vector Transformation){}
      mask Display: disp('L_EB')
  ub,vb,wb : Integrator  InitialCondition=Vm_0  ContinuousStateAttributes=Vm_statename
  xe,ye,ze : Integrator  InitialCondition=xme_0  ContinuousStateAttributes=xme_statename
  Ve : Outport  Unit=m/s  VectorParamsAs1DForOutWhenUnconnected=off
  Xe : Outport  Port=2  Unit=m  VectorParamsAs1DForOutWhenUnconnected=off
  Euler : Outport  Port=3  Unit=rad  VectorParamsAs1DForOutWhenUnconnected=off
  DCM : Outport  Port=4  Unit=1  VectorParamsAs1DForOutWhenUnconnected=off
  Vb : Outport  Port=5  Unit=m/s  VectorParamsAs1DForOutWhenUnconnected=off
  p,q,r : Outport  Port=6  Unit=rad/s  VectorParamsAs1DForOutWhenUnconnected=off
  pdot,qdot,rdot : Outport  Port=7  Unit=rad/s^2  VectorParamsAs1DForOutWhenUnconnected=off
  Ab : Outport  Port=8  Unit=m/s^2  VectorParamsAs1DForOutWhenUnconnected=off
  drone_mass_variable : Outport  Port=9
  wires:
  "Determine Force, Mass & Inertia"/3("I, I_dot ") -> Calculate omega_dot/2
  Calculate DCM & Euler Angles/2 -> Euler/1
  Vbxw/1 -> Sum/2
  xe,ye,ze/1 -> Xe/1
  "transform to Inertial axes "/1(Ve) -> Velocity Conversion1/1(in), xe,ye,ze/1
  "p,q,r "/1 -> Vbxw/2, p,q,r/1, Calculate omega_dot/1, Calculate DCM & Euler Angles/1
  Moments/1 -> Calculate omega_dot/3
  Forces/1 -> "Determine Force, Mass & Inertia"/2(forces)
  Product/1 -> Abi/1, Sum/1
  Calculate DCM & Euler Angles/1 -> DCM/1, Transpose/1
  Transpose/1 -> "transform to Inertial axes "/2(transform coefficients)
  mass/1 -> "Determine Force, Mass & Inertia"/3("mass ")
  "Determine Force, Mass & Inertia"/2(mass) -> Product/2, drone_mass_variable/1
  m_dot/1 -> "Determine Force, Mass & Inertia"/4(mdot)
  "Determine Force, Mass & Inertia"/4(Out9) -> Out9/1
  Calculate omega_dot/1 -> pdot,qdot,rdot/1, "p,q,r "/1
  I/1 -> "Determine Force, Mass & Inertia"/5(I)
  I_dot/1 -> "Determine Force, Mass & Inertia"/6(I_dot)
  "Determine Force, Mass & Inertia"/1("forces ") -> Product/1
  ub,vb,wb/1 -> "Determine Force, Mass & Inertia"/1(Vb), Velocity Conversion/1(in), Vbxw/1, "transform to Inertial axes "/1(x y z)
  Velocity Conversion/1(out) -> Vb/1
  Sum/1 -> ub,vb,wb/1, Ab/1
  Velocity Conversion1/1(out) -> Ve/1
  Vre/1 -> Velocity Conversion2/1

== system SiMoDronesMK/Mass Change Model/Model/Payload + oscillations  ==
  Add : Sum
  Digital Clock : DigitalClock
  First-Order Hold : simulink_need_slupdate/First-Order Hold  DisableCoverage=on  Ts=0.1
      settings: SourceProductBaseCode=SL
  Loaded : Constant  Value=mass
  Loaded1 : Constant  Value=0
  Switch : Switch  Criteria=u2 > Threshold  SaturateOnIntegerOverflow=off  InputSameDT=off
  Uniform Random Number : UniformRandomNumber  Minimum=-(drone.mtot+mass)/50  Maximum=(drone.mtot+mass)/50  SampleTime=0.5
  Payload mass : Outport
  wires:
  Loaded/1 -> Add/1
  Add/1 -> Payload mass/1
  Loaded1/1 -> Switch/1
  Switch/1 -> Add/2
  Digital Clock/1 -> Switch/2
  Uniform Random Number/1 -> First-Order Hold/1
  First-Order Hold/1 -> Switch/3

== system SiMoDronesMK/Mass Change Model/Model/Quad rotor model1 ==
  w : Inport
  Angle_p q r : Inport  Port=2
  vel2 : Inport  Port=3
  drone_mass_variable : Inport  Port=4
  Demux : Demux
  Demux1 : Demux
  Modèle Forces : Subsystem
  Modèle Moments : Subsystem
  F : Outport
  M : Outport  Port=2
  wires:
  w/1 -> Demux/1, Demux1/1  "Propellers Speed"
  Demux/1 -> Modèle Forces/1(In1)
  Demux/4 -> Modèle Forces/4(In4)
  Demux/2 -> Modèle Forces/2(In2)
  Demux/3 -> Modèle Forces/3(In3)
  Demux1/1 -> Modèle Moments/1(In1)
  Demux1/2 -> Modèle Moments/2(In2)
  Demux1/4 -> Modèle Moments/4(In4)
  Demux1/3 -> Modèle Moments/3(In3)
  vel2/1 -> Modèle Forces/5(vel1)  "vel_Rb"
  Angle_p q r/1 -> Modèle Moments/5(vel1)  "p,q,r"
  Modèle Forces/1(Out1) -> F/1  "F_Rb"
  Modèle Moments/1(M) -> M/1  "M_Rb"
  drone_mass_variable/1 -> Modèle Forces/6(drone_mass_variable)

== system SiMoDronesMK/Mass Change Model/Model/Vitesse&Position_Saturation ==
  In1 : Inport
  Compare To Constant : simulink/Logic and Bit Operations/Compare To Constant  relop=<=  const=-0.1  OutDataTypeStr=boolean
  Compare To Zero : simulink/Logic and Bit Operations/Compare To Zero  relop===  OutDataTypeStr=boolean
  Compare To Zero1 : simulink/Logic and Bit Operations/Compare To Zero  relop=>  OutDataTypeStr=boolean
  Demux1 : Demux  Outputs=3
  Demux2 : Demux  Outputs=3
  Display : Display
  Display1 : Display
  Integrator1 : Integrator  InitialCondition=init_state.Pterre0(2)  UpperSaturationLimit=[Inf Inf 0]
  Integrator2 : Integrator  InitialCondition=init_state.Pterre0(1)  UpperSaturationLimit=[Inf Inf 0]
  Integrator3 : Integrator  InitialCondition=init_state.Pterre0(3)  LimitOutput=on  UpperSaturationLimit=[0]
  Logical Operator : Logic  Operator=NAND  AllPortsSameDT=off  OutDataTypeStr=boolean
  Mux : Mux  Inputs=3
  Mux1 : Mux  Inputs=3
  Product : Product  RndMeth=Zero
  Product1 : Product  RndMeth=Zero
  Product2 : Product  RndMeth=Zero
  Ve (m/s) : Outport
  Xe (m) : Outport  Port=2
  wires:
  Compare To Zero1/1 -> Logical Operator/1
  Compare To Zero/1 -> Logical Operator/2
  Demux1/1 -> Mux/1
  Demux1/2 -> Mux/2
  Logical Operator/1 -> Product/2
  Demux1/3 -> Mux/3, Compare To Zero1/1
  In1/1 -> Demux1/1, Demux2/1  "vel"
  Mux/1 -> Product/1  "Vitesse [m/s]"
  Product/1 -> Ve (m/s)/1
  Integrator1/1 -> Mux1/2
  Demux2/3 -> Integrator3/1
  Integrator3/1 -> Display1/1, Compare To Constant/1, Compare To Zero/1, Mux1/3
  Integrator2/1 -> Mux1/1
  Product1/1 -> Integrator2/1
  Demux2/1 -> Product1/1
  Product2/1 -> Integrator1/1
  Demux2/2 -> Product2/1
  Compare To Constant/1 -> Product1/2, Display/1, Product2/2
  Mux1/1 -> Xe (m)/1

== system SiMoDronesMK/Mass Change Model/Model/bus selector ==
  actuators : Inport
  Bus Selector1 : BusSelector  OutputSignals=motor1.current,motor2.current,motor3.current,motor4.current
  Bus Selector2 : BusSelector  OutputSignals=motor1.speed,motor2.speed,motor3.speed,motor4.speed
  Bus Selector3 : BusSelector  OutputSignals=motor1.current,motor2.current,motor3.current,motor4.current
  Mux : Mux
  Mux1 : Mux
  Sum : Sum  Inputs=++++
  Total current : Outport
  currents : Outport  Port=2
  prop speed : Outport  Port=3
  wires:
  Bus Selector3/3 -> Mux1/3  "<current>"
  Bus Selector3/4 -> Mux1/4  "<current>"
  Bus Selector3/1 -> Mux1/1  "<current>"
  Bus Selector3/2 -> Mux1/2  "<current>"
  Mux1/1 -> currents/1
  Bus Selector2/3 -> Mux/3  "<speed>"
  Bus Selector2/4 -> Mux/4  "<speed>"
  Bus Selector2/1 -> Mux/1  "<speed>"
  Bus Selector2/2 -> Mux/2  "<speed>"
  Mux/1 -> prop speed/1
  Bus Selector1/3 -> Sum/3  "<current>"
  Bus Selector1/4 -> Sum/4  "<current>"
  Bus Selector1/1 -> Sum/1  "<current>"
  Bus Selector1/2 -> Sum/2  "<current>"
  actuators/1 -> Bus Selector1/1, Bus Selector2/1, Bus Selector3/1
  Sum/1 -> Total current/1
